simulink model "proba1"  (Simulink 7.0)
settings: Solver=ode1  StartTime=0.0  StopTime=Inf  FixedStep=0.001  RelTol=1e-3
PostLoadFcn:
  | ,try, rti_mdl_postloadfcn(bdroot, 'UpdateModel', 280, 'rti1005'); catch, disp(lasterr); end,
libraries: simulink x23, simulink_extras x10, rtilibm x8
(part 2 of 2)

== system proba1/serwomechanizmy/os6/ograniczenie3 ==
  In1 : Inport
  Compare To Constant : simulink/Logic and Bit Operations/Compare To Constant  SystemSampleTime=-1  relop=<=  const=890  LogicOutDataTypeMode=boolean  ZeroCross=off
  Compare To Constant1 : simulink/Logic and Bit Operations/Compare To Constant  SystemSampleTime=-1  relop=>=  const=0  LogicOutDataTypeMode=boolean  ZeroCross=off
  Constant1 : Constant  Value=0
  Logical Operator : Logic  AllPortsSameDT=off  OutDataTypeMode=boolean
  Switch : Switch  Criteria=u2 ~= 0
  Out1 : Outport
  wires:
  In1/1 -> Compare To Constant/1, Compare To Constant1/1, Switch/1
  Compare To Constant1/1 -> Logical Operator/1
  Compare To Constant/1 -> Logical Operator/2
  Logical Operator/1 -> Switch/2
  Constant1/1 -> Switch/3
  Switch/1 -> Out1/1

== system proba1/serwomechanizmy/os6/skalowanie ==
  In1 : Inport
  Fcn : Fcn  Expr=(u(1)*(2^23)*pi())/1000
  Gain2 : Gain  Gain=1.25/pi()
  Out1 : Outport
  wires:
  Fcn/1 -> Gain2/1
  Gain2/1 -> Out1/1
  In1/1 -> Fcn/1

== system proba1/tryby/kinematyka odwrotna/podaj wyliczone wartosci ==
  obliczoneFi1 : Inport
  obliczoneFi2 : Inport  Port=2
  ObliczoneFi3 : Inport  Port=3
  Enable : EnablePort
  Data Store Write : DataStoreWrite  DataStoreName=obliczoneFi1  SampleTime=-1
  Data Store Write1 : DataStoreWrite  DataStoreName=obliczoneFi2  SampleTime=-1
  Data Store Write2 : DataStoreWrite  DataStoreName=obliczoneFi3  SampleTime=-1
  wires:
  obliczoneFi1/1 -> Data Store Write/1
  obliczoneFi2/1 -> Data Store Write1/1
  ObliczoneFi3/1 -> Data Store Write2/1

== system proba1/tryby/rozpoznawanie obrazu/podaj wyliczone wartosci ==
  zadaneX : Inport
  zadaneY : Inport  Port=2
  zadaneZ : Inport  Port=3
  Data Store Write : DataStoreWrite  DataStoreName=ObliczoneX  SampleTime=-1
  Data Store Write1 : DataStoreWrite  DataStoreName=ObliczoneY  SampleTime=-1
  Data Store Write2 : DataStoreWrite  DataStoreName=ObliczoneZ  SampleTime=-1
  wires:
  zadaneX/1 -> Data Store Write/1
  zadaneY/1 -> Data Store Write1/1
  zadaneZ/1 -> Data Store Write2/1

== system proba1/RTI Data/RTI Data Store/RTI Data Store/RTI Data Store ==
  RTI Data Store : Subsystem
      mask Type: RTI_DATA_STORE
      mask Description:
      | RTI Data Store Block. This block is used by RTI to store internal model dependent data. Deleting this block will result in data loss.
      | 
      | NEVER DELETE, COPY, OR MODIFY THIS BLOCK!
      mask Help:
      | RTI Data Store Block. This block is used by RTI to store internal model dependent data. Deleting this block will result in data loss.
      | 
      | NEVER DELETE, COPY, OR MODIFY THIS BLOCK!
      mask Display: text(0.5, 0.5, ' ', 'HorizontalAlignment', 'center');

== system proba1/serwomechanizmy/os1/Position 1/Filters 1 ==
  Sin && Cos : Inport
  Analog Butterworth LP Filter : Subsystem  mask(buttap){@1=2*pi*16, @2=1}
      mask prompts: @1 "Cutoff frequency (rad/sec)"; @2 "Order"
      mask help:
      | Analog Butterworth low pass filter.
      |
      | (Requires Signal Processing Toolbox)
      mask init:
      | [z,p,k]=buttap(@2); z=@1*z; p=@1*p; k=real(prod(-p)); [num,den]=zp2tf(z,p,k); w=logspace(log10(@1/10),log10(10*@1),20); h=freqs(num,den,w);
      mask Help: Butterworth low pass filter using MATLAB's butter command.
      mask Display: plot(20*log10(w),20*log10(abs(h)))
  Analog Butterworth LP Filter1 : Subsystem  mask(buttap){@1=2*pi*16, @2=1}
      mask prompts: @1 "Cutoff frequency (rad/sec)"; @2 "Order"
      mask help:
      | Analog Butterworth low pass filter.
      |
      | (Requires Signal Processing Toolbox)
      mask init:
      | [z,p,k]=buttap(@2); z=@1*z; p=@1*p; k=real(prod(-p)); [num,den]=zp2tf(z,p,k); w=logspace(log10(@1/10),log10(10*@1),20); h=freqs(num,den,w);
      mask Help: Butterworth low pass filter using MATLAB's butter command.
      mask Display: plot(20*log10(w),20*log10(abs(h)))
  Demux : Demux  Outputs=2
  Sin : Outport
  Cos : Outport  Port=2
  wires:
  Demux/2 -> Analog Butterworth LP Filter1/1(In1)
  Demux/1 -> Analog Butterworth LP Filter/1(In1)
  Sin && Cos/1 -> Demux/1
  Analog Butterworth LP Filter1/1(Out1) -> Cos/1
  Analog Butterworth LP Filter/1(Out1) -> Sin/1

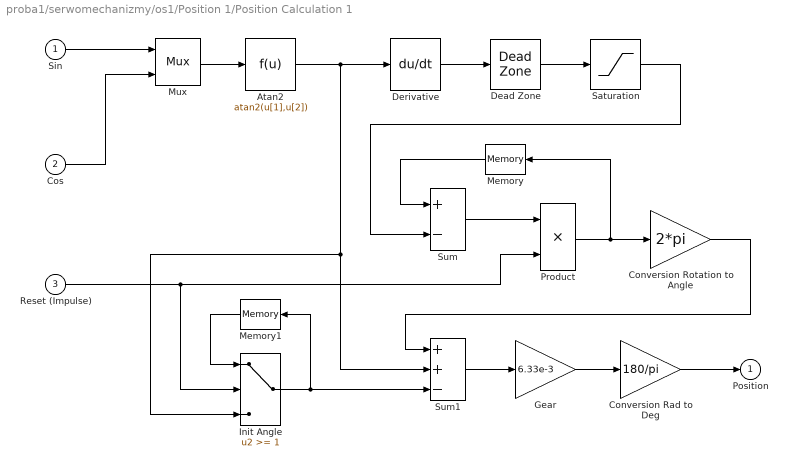
== system proba1/serwomechanizmy/os1/Position 1/Position Calculation 1 ==
  Sin : Inport
  Cos : Inport  Port=2
  Reset (Impulse) : Inport  Port=3
  Atan2 : Fcn  Expr=atan2(u[1],u[2])
  Conversion Rad to Deg : Gain  Gain=180/pi  SaturateOnIntegerOverflow=on
  Conversion Rotation to Angle : Gain  Gain=2*pi  SaturateOnIntegerOverflow=on
  Dead Zone : DeadZone  LowerValue=-5000  UpperValue=5000  SaturateOnIntegerOverflow=on
  Derivative : Derivative
  Gear : Gain  Gain=6.33e-3  SaturateOnIntegerOverflow=on
  Init Angle : Switch  Threshold=1  SaturateOnIntegerOverflow=on  InputSameDT=on
  Memory : Memory  Orientation=left
  Memory1 : Memory  Orientation=left
  Mux : Mux  Inputs=2
  Product : Product  SaturateOnIntegerOverflow=on  RndMeth=Zero  InputSameDT=on
  Saturation : Saturate  UpperLimit=1  LowerLimit=-1
  Sum : Sum  Inputs=+-  SaturateOnIntegerOverflow=on  InputSameDT=on
  Sum1 : Sum  Inputs=++-  SaturateOnIntegerOverflow=on  InputSameDT=on
  Position : Outport
  wires:
  Init Angle/1 -> Memory1/1, Sum1/3
  Memory1/1 -> Init Angle/1
  Product/1 -> Memory/1, Conversion Rotation to Angle/1
  Memory/1 -> Sum/1
  Cos/1 -> Mux/2
  Atan2/1 -> Init Angle/3, Sum1/2, Derivative/1
  Reset (Impulse)/1 -> Init Angle/2, Product/2
  Conversion Rotation to Angle/1 -> Sum1/1
  Saturation/1 -> Sum/2
  Conversion Rad to Deg/1 -> Position/1
  Sin/1 -> Mux/1
  Mux/1 -> Atan2/1
  Derivative/1 -> Dead Zone/1
  Dead Zone/1 -> Saturation/1
  Sum/1 -> Product/1
  Sum1/1 -> Gear/1
  Gear/1 -> Conversion Rad to Deg/1

== system proba1/serwomechanizmy/os1/blok bazowania/zerowanie ==
  Enable : EnablePort
  Constant : Constant  Value=0
  Data Store Write : DataStoreWrite  DataStoreName=u1  SampleTime=-1
  Data Store Write1 : DataStoreWrite  DataStoreName=tmp_u1  SampleTime=-1
  wires:
  Constant/1 -> Data Store Write/1, Data Store Write1/1

== system proba1/serwomechanizmy/os2/Position 2/Filters 2 ==
  Sin && Cos : Inport
  Analog Butterworth LP Filter : Subsystem  mask(buttap){@1=2*pi*16, @2=1}
      mask prompts: @1 "Cutoff frequency (rad/sec)"; @2 "Order"
      mask help:
      | Analog Butterworth low pass filter.
      |
      | (Requires Signal Processing Toolbox)
      mask init:
      | [z,p,k]=buttap(@2); z=@1*z; p=@1*p; k=real(prod(-p)); [num,den]=zp2tf(z,p,k); w=logspace(log10(@1/10),log10(10*@1),20); h=freqs(num,den,w);
      mask Help: Butterworth low pass filter using MATLAB's butter command.
      mask Display: plot(20*log10(w),20*log10(abs(h)))
  Analog Butterworth LP Filter1 : Subsystem  mask(buttap){@1=2*pi*16, @2=1}
      mask prompts: @1 "Cutoff frequency (rad/sec)"; @2 "Order"
      mask help:
      | Analog Butterworth low pass filter.
      |
      | (Requires Signal Processing Toolbox)
      mask init:
      | [z,p,k]=buttap(@2); z=@1*z; p=@1*p; k=real(prod(-p)); [num,den]=zp2tf(z,p,k); w=logspace(log10(@1/10),log10(10*@1),20); h=freqs(num,den,w);
      mask Help: Butterworth low pass filter using MATLAB's butter command.
      mask Display: plot(20*log10(w),20*log10(abs(h)))
  Demux : Demux  Outputs=2
  Sin : Outport
  Cos : Outport  Port=2
  wires:
  Demux/2 -> Analog Butterworth LP Filter1/1(In1)
  Demux/1 -> Analog Butterworth LP Filter/1(In1)
  Sin && Cos/1 -> Demux/1
  Analog Butterworth LP Filter1/1(Out1) -> Cos/1
  Analog Butterworth LP Filter/1(Out1) -> Sin/1

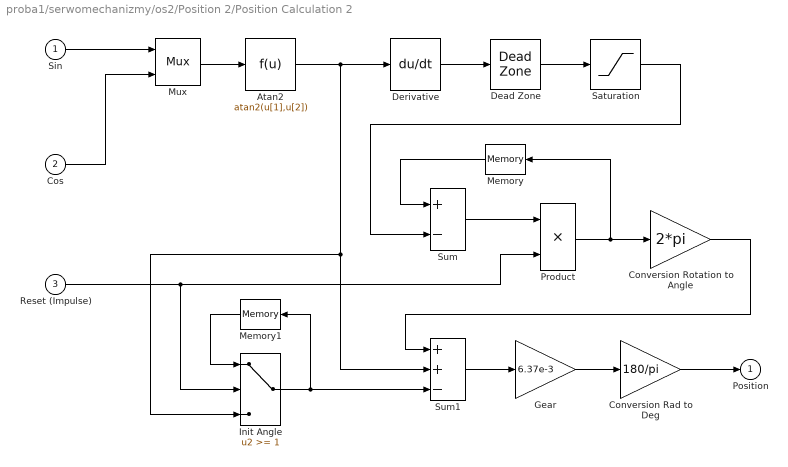
== system proba1/serwomechanizmy/os2/Position 2/Position Calculation 2 ==
  Sin : Inport
  Cos : Inport  Port=2
  Reset (Impulse) : Inport  Port=3
  Atan2 : Fcn  Expr=atan2(u[1],u[2])
  Conversion Rad to Deg : Gain  Gain=180/pi  SaturateOnIntegerOverflow=on
  Conversion Rotation to Angle : Gain  Gain=2*pi  SaturateOnIntegerOverflow=on
  Dead Zone : DeadZone  LowerValue=-5000  UpperValue=5000  SaturateOnIntegerOverflow=on
  Derivative : Derivative
  Gear : Gain  Gain=6.37e-3  SaturateOnIntegerOverflow=on
  Init Angle : Switch  Threshold=1  SaturateOnIntegerOverflow=on  InputSameDT=on
  Memory : Memory  Orientation=left
  Memory1 : Memory  Orientation=left
  Mux : Mux  Inputs=2
  Product : Product  SaturateOnIntegerOverflow=on  RndMeth=Zero  InputSameDT=on
  Saturation : Saturate  UpperLimit=1  LowerLimit=-1
  Sum : Sum  Inputs=+-  SaturateOnIntegerOverflow=on  InputSameDT=on
  Sum1 : Sum  Inputs=++-  SaturateOnIntegerOverflow=on  InputSameDT=on
  Position : Outport
  wires:
  Init Angle/1 -> Memory1/1, Sum1/3
  Memory1/1 -> Init Angle/1
  Product/1 -> Memory/1, Conversion Rotation to Angle/1
  Memory/1 -> Sum/1
  Cos/1 -> Mux/2
  Atan2/1 -> Init Angle/3, Sum1/2, Derivative/1
  Reset (Impulse)/1 -> Init Angle/2, Product/2
  Conversion Rotation to Angle/1 -> Sum1/1
  Saturation/1 -> Sum/2
  Conversion Rad to Deg/1 -> Position/1
  Sin/1 -> Mux/1
  Mux/1 -> Atan2/1
  Derivative/1 -> Dead Zone/1
  Dead Zone/1 -> Saturation/1
  Sum/1 -> Product/1
  Sum1/1 -> Gear/1
  Gear/1 -> Conversion Rad to Deg/1

== system proba1/serwomechanizmy/os2/blok bazowania/zerowanie ==
  Enable : EnablePort
  Constant : Constant  Value=0
  Data Store Write : DataStoreWrite  DataStoreName=u2  SampleTime=-1
  Data Store Write1 : DataStoreWrite  DataStoreName=tmp_u2  SampleTime=-1
  wires:
  Constant/1 -> Data Store Write/1, Data Store Write1/1

== system proba1/serwomechanizmy/os3/Position 3/Filters 3 ==
  Sin && Cos : Inport
  Analog Butterworth LP Filter : Subsystem  mask(buttap){@1=2*pi*16, @2=1}
      mask prompts: @1 "Cutoff frequency (rad/sec)"; @2 "Order"
      mask help:
      | Analog Butterworth low pass filter.
      |
      | (Requires Signal Processing Toolbox)
      mask init:
      | [z,p,k]=buttap(@2); z=@1*z; p=@1*p; k=real(prod(-p)); [num,den]=zp2tf(z,p,k); w=logspace(log10(@1/10),log10(10*@1),20); h=freqs(num,den,w);
      mask Help: Butterworth low pass filter using MATLAB's butter command.
      mask Display: plot(20*log10(w),20*log10(abs(h)))
  Analog Butterworth LP Filter1 : Subsystem  mask(buttap){@1=2*pi*16, @2=1}
      mask prompts: @1 "Cutoff frequency (rad/sec)"; @2 "Order"
      mask help:
      | Analog Butterworth low pass filter.
      |
      | (Requires Signal Processing Toolbox)
      mask init:
      | [z,p,k]=buttap(@2); z=@1*z; p=@1*p; k=real(prod(-p)); [num,den]=zp2tf(z,p,k); w=logspace(log10(@1/10),log10(10*@1),20); h=freqs(num,den,w);
      mask Help: Butterworth low pass filter using MATLAB's butter command.
      mask Display: plot(20*log10(w),20*log10(abs(h)))
  Demux : Demux  Outputs=2
  Sin : Outport
  Cos : Outport  Port=2
  wires:
  Demux/2 -> Analog Butterworth LP Filter1/1(In1)
  Demux/1 -> Analog Butterworth LP Filter/1(In1)
  Sin && Cos/1 -> Demux/1
  Analog Butterworth LP Filter1/1(Out1) -> Cos/1
  Analog Butterworth LP Filter/1(Out1) -> Sin/1

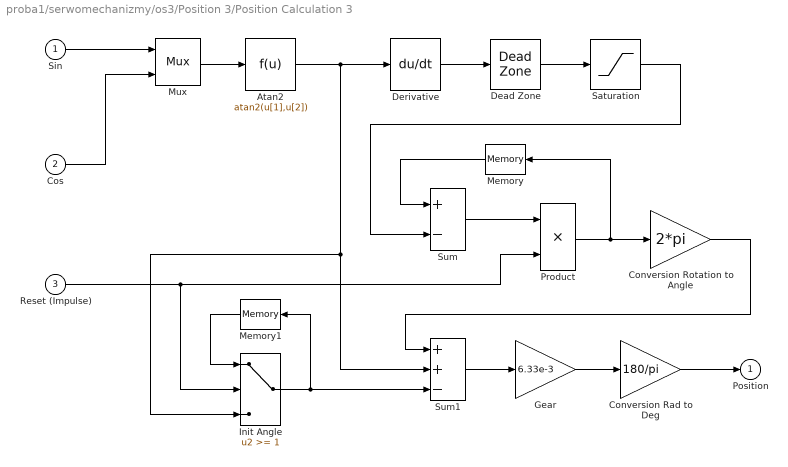
== system proba1/serwomechanizmy/os3/Position 3/Position Calculation 3 ==
  Sin : Inport
  Cos : Inport  Port=2
  Reset (Impulse) : Inport  Port=3
  Atan2 : Fcn  Expr=atan2(u[1],u[2])
  Conversion Rad to Deg : Gain  Gain=180/pi  SaturateOnIntegerOverflow=on
  Conversion Rotation to Angle : Gain  Gain=2*pi  SaturateOnIntegerOverflow=on
  Dead Zone : DeadZone  LowerValue=-5000  UpperValue=5000  SaturateOnIntegerOverflow=on
  Derivative : Derivative
  Gear : Gain  Gain=6.33e-3  SaturateOnIntegerOverflow=on
  Init Angle : Switch  Threshold=1  SaturateOnIntegerOverflow=on  InputSameDT=on
  Memory : Memory  Orientation=left
  Memory1 : Memory  Orientation=left
  Mux : Mux  Inputs=2
  Product : Product  SaturateOnIntegerOverflow=on  RndMeth=Zero  InputSameDT=on
  Saturation : Saturate  UpperLimit=1  LowerLimit=-1
  Sum : Sum  Inputs=+-  SaturateOnIntegerOverflow=on  InputSameDT=on
  Sum1 : Sum  Inputs=++-  SaturateOnIntegerOverflow=on  InputSameDT=on
  Position : Outport
  wires:
  Init Angle/1 -> Memory1/1, Sum1/3
  Memory1/1 -> Init Angle/1
  Product/1 -> Memory/1, Conversion Rotation to Angle/1
  Memory/1 -> Sum/1
  Cos/1 -> Mux/2
  Atan2/1 -> Init Angle/3, Sum1/2, Derivative/1
  Reset (Impulse)/1 -> Init Angle/2, Product/2
  Conversion Rotation to Angle/1 -> Sum1/1
  Saturation/1 -> Sum/2
  Conversion Rad to Deg/1 -> Position/1
  Sin/1 -> Mux/1
  Mux/1 -> Atan2/1
  Derivative/1 -> Dead Zone/1
  Dead Zone/1 -> Saturation/1
  Sum/1 -> Product/1
  Sum1/1 -> Gear/1
  Gear/1 -> Conversion Rad to Deg/1

== system proba1/serwomechanizmy/os3/blok bazowania/zerowanie ==
  Enable : EnablePort
  Constant : Constant  Value=0
  Data Store Write : DataStoreWrite  DataStoreName=u3  SampleTime=-1
  Data Store Write1 : DataStoreWrite  DataStoreName=tmp_u3  SampleTime=-1
  wires:
  Constant/1 -> Data Store Write/1, Data Store Write1/1

== system proba1/serwomechanizmy/os4/Position 4/Filters 4 ==
  Sin && Cos : Inport
  Analog Butterworth LP Filter : Subsystem  mask(buttap){@1=2*pi*16, @2=1}
      mask prompts: @1 "Cutoff frequency (rad/sec)"; @2 "Order"
      mask help:
      | Analog Butterworth low pass filter.
      |
      | (Requires Signal Processing Toolbox)
      mask init:
      | [z,p,k]=buttap(@2); z=@1*z; p=@1*p; k=real(prod(-p)); [num,den]=zp2tf(z,p,k); w=logspace(log10(@1/10),log10(10*@1),20); h=freqs(num,den,w);
      mask Help: Butterworth low pass filter using MATLAB's butter command.
      mask Display: plot(20*log10(w),20*log10(abs(h)))
  Analog Butterworth LP Filter1 : Subsystem  mask(buttap){@1=2*pi*16, @2=1}
      mask prompts: @1 "Cutoff frequency (rad/sec)"; @2 "Order"
      mask help:
      | Analog Butterworth low pass filter.
      |
      | (Requires Signal Processing Toolbox)
      mask init:
      | [z,p,k]=buttap(@2); z=@1*z; p=@1*p; k=real(prod(-p)); [num,den]=zp2tf(z,p,k); w=logspace(log10(@1/10),log10(10*@1),20); h=freqs(num,den,w);
      mask Help: Butterworth low pass filter using MATLAB's butter command.
      mask Display: plot(20*log10(w),20*log10(abs(h)))
  Demux : Demux  Outputs=2
  Sin : Outport
  Cos : Outport  Port=2
  wires:
  Analog Butterworth LP Filter/1(Out1) -> Sin/1
  Analog Butterworth LP Filter1/1(Out1) -> Cos/1
  Sin && Cos/1 -> Demux/1
  Demux/1 -> Analog Butterworth LP Filter/1(In1)
  Demux/2 -> Analog Butterworth LP Filter1/1(In1)

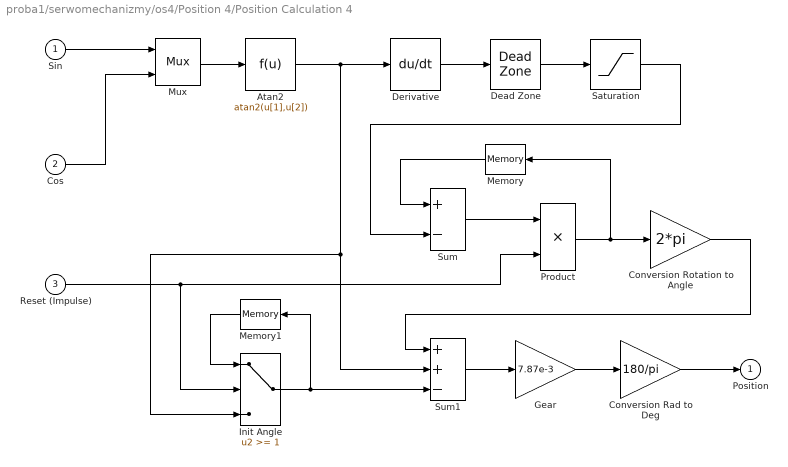
== system proba1/serwomechanizmy/os4/Position 4/Position Calculation 4 ==
  Sin : Inport
  Cos : Inport  Port=2
  Reset (Impulse) : Inport  Port=3
  Atan2 : Fcn  Expr=atan2(u[1],u[2])
  Conversion Rad to Deg : Gain  Gain=180/pi  SaturateOnIntegerOverflow=on
  Conversion Rotation to Angle : Gain  Gain=2*pi  SaturateOnIntegerOverflow=on
  Dead Zone : DeadZone  LowerValue=-5000  UpperValue=5000  SaturateOnIntegerOverflow=on
  Derivative : Derivative
  Gear : Gain  Gain=7.87e-3  SaturateOnIntegerOverflow=on
  Init Angle : Switch  Threshold=1  SaturateOnIntegerOverflow=on  InputSameDT=on
  Memory : Memory  Orientation=left
  Memory1 : Memory  Orientation=left
  Mux : Mux  Inputs=2
  Product : Product  SaturateOnIntegerOverflow=on  RndMeth=Zero  InputSameDT=on
  Saturation : Saturate  UpperLimit=1  LowerLimit=-1
  Sum : Sum  Inputs=+-  SaturateOnIntegerOverflow=on  InputSameDT=on
  Sum1 : Sum  Inputs=++-  SaturateOnIntegerOverflow=on  InputSameDT=on
  Position : Outport
  wires:
  Gear/1 -> Conversion Rad to Deg/1
  Sum1/1 -> Gear/1
  Sum/1 -> Product/1
  Dead Zone/1 -> Saturation/1
  Derivative/1 -> Dead Zone/1
  Mux/1 -> Atan2/1
  Sin/1 -> Mux/1
  Conversion Rad to Deg/1 -> Position/1
  Saturation/1 -> Sum/2
  Conversion Rotation to Angle/1 -> Sum1/1
  Reset (Impulse)/1 -> Product/2, Init Angle/2
  Atan2/1 -> Derivative/1, Sum1/2, Init Angle/3
  Cos/1 -> Mux/2
  Memory/1 -> Sum/1
  Product/1 -> Conversion Rotation to Angle/1, Memory/1
  Memory1/1 -> Init Angle/1
  Init Angle/1 -> Sum1/3, Memory1/1

== system proba1/serwomechanizmy/os5/Position 5/Filters 5 ==
  Sin && Cos : Inport
  Analog Butterworth LP Filter : Subsystem  mask(buttap){@1=2*pi*16, @2=1}
      mask prompts: @1 "Cutoff frequency (rad/sec)"; @2 "Order"
      mask help:
      | Analog Butterworth low pass filter.
      |
      | (Requires Signal Processing Toolbox)
      mask init:
      | [z,p,k]=buttap(@2); z=@1*z; p=@1*p; k=real(prod(-p)); [num,den]=zp2tf(z,p,k); w=logspace(log10(@1/10),log10(10*@1),20); h=freqs(num,den,w);
      mask Help: Butterworth low pass filter using MATLAB's butter command.
      mask Display: plot(20*log10(w),20*log10(abs(h)))
  Analog Butterworth LP Filter1 : Subsystem  mask(buttap){@1=2*pi*16, @2=1}
      mask prompts: @1 "Cutoff frequency (rad/sec)"; @2 "Order"
      mask help:
      | Analog Butterworth low pass filter.
      |
      | (Requires Signal Processing Toolbox)
      mask init:
      | [z,p,k]=buttap(@2); z=@1*z; p=@1*p; k=real(prod(-p)); [num,den]=zp2tf(z,p,k); w=logspace(log10(@1/10),log10(10*@1),20); h=freqs(num,den,w);
      mask Help: Butterworth low pass filter using MATLAB's butter command.
      mask Display: plot(20*log10(w),20*log10(abs(h)))
  Demux : Demux  Outputs=2
  Sin : Outport
  Cos : Outport  Port=2
  wires:
  Analog Butterworth LP Filter/1(Out1) -> Sin/1
  Analog Butterworth LP Filter1/1(Out1) -> Cos/1
  Sin && Cos/1 -> Demux/1
  Demux/1 -> Analog Butterworth LP Filter/1(In1)
  Demux/2 -> Analog Butterworth LP Filter1/1(In1)

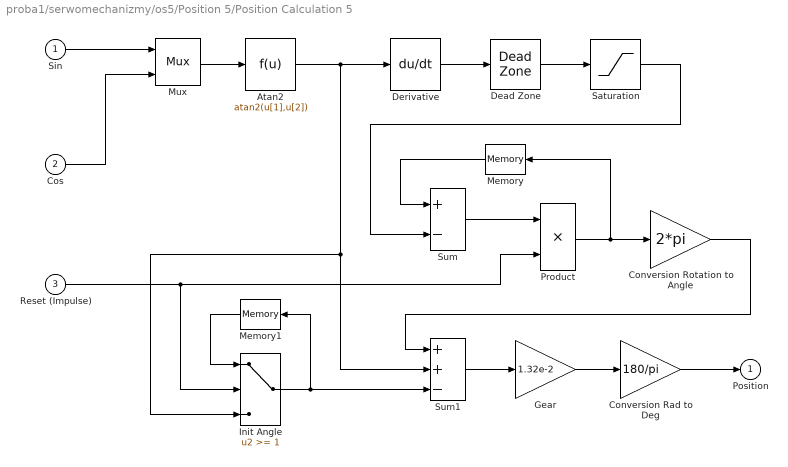
== system proba1/serwomechanizmy/os5/Position 5/Position Calculation 5 ==
  Sin : Inport
  Cos : Inport  Port=2
  Reset (Impulse) : Inport  Port=3
  Atan2 : Fcn  Expr=atan2(u[1],u[2])
  Conversion Rad to Deg : Gain  Gain=180/pi  SaturateOnIntegerOverflow=on
  Conversion Rotation to Angle : Gain  Gain=2*pi  SaturateOnIntegerOverflow=on
  Dead Zone : DeadZone  LowerValue=-5000  UpperValue=5000  SaturateOnIntegerOverflow=on
  Derivative : Derivative
  Gear : Gain  Gain=1.32e-2  SaturateOnIntegerOverflow=on
  Init Angle : Switch  Threshold=1  SaturateOnIntegerOverflow=on  InputSameDT=on
  Memory : Memory  Orientation=left
  Memory1 : Memory  Orientation=left
  Mux : Mux  Inputs=2
  Product : Product  SaturateOnIntegerOverflow=on  RndMeth=Zero  InputSameDT=on
  Saturation : Saturate  UpperLimit=1  LowerLimit=-1
  Sum : Sum  Inputs=+-  SaturateOnIntegerOverflow=on  InputSameDT=on
  Sum1 : Sum  Inputs=++-  SaturateOnIntegerOverflow=on  InputSameDT=on
  Position : Outport
  wires:
  Gear/1 -> Conversion Rad to Deg/1
  Sum1/1 -> Gear/1
  Sum/1 -> Product/1
  Dead Zone/1 -> Saturation/1
  Derivative/1 -> Dead Zone/1
  Mux/1 -> Atan2/1
  Sin/1 -> Mux/1
  Conversion Rad to Deg/1 -> Position/1
  Saturation/1 -> Sum/2
  Conversion Rotation to Angle/1 -> Sum1/1
  Reset (Impulse)/1 -> Product/2, Init Angle/2
  Atan2/1 -> Derivative/1, Sum1/2, Init Angle/3
  Cos/1 -> Mux/2
  Memory/1 -> Sum/1
  Product/1 -> Conversion Rotation to Angle/1, Memory/1
  Memory1/1 -> Init Angle/1
  Init Angle/1 -> Sum1/3, Memory1/1

== system proba1/serwomechanizmy/os6/blok bazowania/zerowanie ==
  Enable : EnablePort
  Constant : Constant  Value=0
  Data Store Write : DataStoreWrite  DataStoreName=u4  SampleTime=-1
  Data Store Write1 : DataStoreWrite  DataStoreName=tmp_u4  SampleTime=-1
  wires:
  Constant/1 -> Data Store Write/1, Data Store Write1/1

== system proba1/RTI Data/RTI Data Store/RTI Data Store/RTI Data Store/RTI Data Store ==

== system proba1/serwomechanizmy/os1/Position 1/Filters 1/Analog Butterworth LP Filter ==
  In1 : Inport
  Analog Butterworth LP Filter : ZeroPole  Zeros=z  Poles=p  Gain=k
  Out1 : Outport
  wires:
  Analog Butterworth LP Filter/1 -> Out1/1
  In1/1 -> Analog Butterworth LP Filter/1

== system proba1/serwomechanizmy/os1/Position 1/Filters 1/Analog Butterworth LP Filter1 ==
  In1 : Inport
  Analog Butterworth LP Filter1 : ZeroPole  Zeros=z  Poles=p  Gain=k
  Out1 : Outport
  wires:
  Analog Butterworth LP Filter1/1 -> Out1/1
  In1/1 -> Analog Butterworth LP Filter1/1

== system proba1/serwomechanizmy/os2/Position 2/Filters 2/Analog Butterworth LP Filter ==
  In1 : Inport
  Analog Butterworth LP Filter : ZeroPole  Zeros=z  Poles=p  Gain=k
  Out1 : Outport
  wires:
  Analog Butterworth LP Filter/1 -> Out1/1
  In1/1 -> Analog Butterworth LP Filter/1

== system proba1/serwomechanizmy/os2/Position 2/Filters 2/Analog Butterworth LP Filter1 ==
  In1 : Inport
  Analog Butterworth LP Filter1 : ZeroPole  Zeros=z  Poles=p  Gain=k
  Out1 : Outport
  wires:
  Analog Butterworth LP Filter1/1 -> Out1/1
  In1/1 -> Analog Butterworth LP Filter1/1

== system proba1/serwomechanizmy/os3/Position 3/Filters 3/Analog Butterworth LP Filter ==
  In1 : Inport
  Analog Butterworth LP Filter : ZeroPole  Zeros=z  Poles=p  Gain=k
  Out1 : Outport
  wires:
  Analog Butterworth LP Filter/1 -> Out1/1
  In1/1 -> Analog Butterworth LP Filter/1

== system proba1/serwomechanizmy/os3/Position 3/Filters 3/Analog Butterworth LP Filter1 ==
  In1 : Inport
  Analog Butterworth LP Filter1 : ZeroPole  Zeros=z  Poles=p  Gain=k
  Out1 : Outport
  wires:
  Analog Butterworth LP Filter1/1 -> Out1/1
  In1/1 -> Analog Butterworth LP Filter1/1

== system proba1/serwomechanizmy/os4/Position 4/Filters 4/Analog Butterworth LP Filter ==
  In1 : Inport
  Analog Butterworth LP Filter : ZeroPole  Zeros=z  Poles=p  Gain=k
  Out1 : Outport
  wires:
  Analog Butterworth LP Filter/1 -> Out1/1
  In1/1 -> Analog Butterworth LP Filter/1

== system proba1/serwomechanizmy/os4/Position 4/Filters 4/Analog Butterworth LP Filter1 ==
  In1 : Inport
  Analog Butterworth LP Filter1 : ZeroPole  Zeros=z  Poles=p  Gain=k
  Out1 : Outport
  wires:
  Analog Butterworth LP Filter1/1 -> Out1/1
  In1/1 -> Analog Butterworth LP Filter1/1

== system proba1/serwomechanizmy/os5/Position 5/Filters 5/Analog Butterworth LP Filter ==
  In1 : Inport
  Analog Butterworth LP Filter : ZeroPole  Zeros=z  Poles=p  Gain=k
  Out1 : Outport
  wires:
  Analog Butterworth LP Filter/1 -> Out1/1
  In1/1 -> Analog Butterworth LP Filter/1

== system proba1/serwomechanizmy/os5/Position 5/Filters 5/Analog Butterworth LP Filter1 ==
  In1 : Inport
  Analog Butterworth LP Filter1 : ZeroPole  Zeros=z  Poles=p  Gain=k
  Out1 : Outport
  wires:
  Analog Butterworth LP Filter1/1 -> Out1/1
  In1/1 -> Analog Butterworth LP Filter1/1

== matlab function tryby/rozpoznawanie obrazu/Embedded MATLAB Function ==
  data: x output inherited; y output inherited; z output inherited
function [x, y, z] = fcn()
% This block supports the Embedded MATLAB subset.
% See the help menu for details. 
x = 700;
y = 200;
z = 1100;
